simulink model "DefaultTransitiontoJunction"  (R2020b)
settings: Solver=VariableStepAuto  StartTime=0.0  StopTime=10.0  RelTol=1e-3
settings Model: Creator=apple  LastModifiedBy=apple

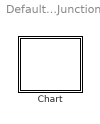
== system DefaultTransitiontoJunction ==
  Chart : Stateflow chart  TreatAsAtomicUnit=on

== stateflow chart DefaultTransitiontoJunction/Chart ==
  state B
    en:fprintf("Entry B");
    du:fprintf("During B");
    ex:fprintf("Exit B");
    state B2
      en:fprintf("Entry B2");
      du:fprintf("During B2");
      ex:fprintf("Exit B2");
    state B1
      en:fprintf("Entry B1");
      du:fprintf("During B1");
      ex:fprintf("Exit B1");
    (default) -> (junction 8)
    (junction 8) -> B2 [order 1] : [x>0]
    (junction 8) -> B1 [order 2]
  state A
    en:fprintf("Entry A");
    du:fprintf("During A");
    ex:fprintf("Exit A");
  (default) -> A : {x= 0;}
  A -> B : E_one/{fprintf("Transition Action");}
  data: x local
  events: E_one local FUNCTION_CALL_EVENT
